simulink model "lab2_sim"  (R2019b)
settings: Solver=ode45  StartTime=0.0  StopTime=Tfin  MaxStep=Tstep  RelTol=1e-3
values from neighbouring files (symbols this model uses):
  C = [1, 0, 0]    [lab2_prac.m]
  K = place(AAA, BBB, [-1, -20, -3])    [lab2_prac.m]
  u_bar = 0    [lab2_prac.m]
  x0 = [0, 0, 0]    [lab2_prac.m]
  x_bar = [1, 0, 0]    [lab2_prac.m]
settings Model: Creator=user  LastModifiedBy=user

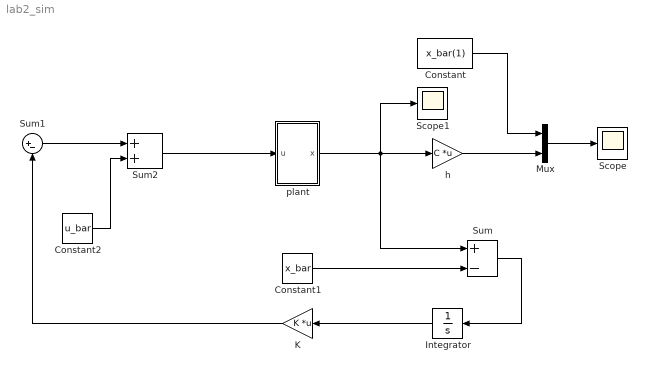
== system lab2_sim ==
  Constant : Constant  Value=x_bar(1)
  Constant1 : Constant  Value=x_bar
  Constant2 : Constant  Value=u_bar
  Integrator : Integrator
  K : Gain  Gain=K  Multiplication=Matrix(K*u)
  Mux : Mux  Inputs=2
  Scope : Scope
  Scope1 : Scope
  Sum : Sum  Inputs=+-
  Sum1 : Sum  Inputs=|+-
  Sum2 : Sum
  h : Gain  Gain=C  Multiplication=Matrix(K*u)
  plant : Subsystem
  wires:
  plant/1(x) -> Scope1/1, Sum/1, h/1
  h/1 -> Mux/2
  Mux/1 -> Scope/1
  Constant/1 -> Mux/1
  Constant1/1 -> Sum/2
  Sum/1 -> Integrator/1
  K/1 -> Sum1/2
  Sum1/1 -> Sum2/1
  Sum2/1 -> plant/1(u)
  Constant2/1 -> Sum2/2
  Integrator/1 -> K/1

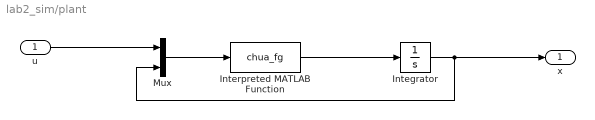
== system lab2_sim/plant ==
  u : Inport
  Integrator : Integrator  InitialCondition=x0
  Interpreted MATLAB Function : MATLABFcn  MATLABFcn=chua_fg
  Mux : Mux  Inputs=2
  x : Outport
  wires:
  Mux/1 -> Interpreted MATLAB Function/1
  Integrator/1 -> x/1, Mux/2
  u/1 -> Mux/1
  Interpreted MATLAB Function/1 -> Integrator/1
